simulink model "rudder_calibration"  (Simulink 7.5)
settings: Solver=FixedStepDiscrete  SolverMode=SingleTasking  StartTime=0.0  StopTime=10.0  FixedStep=0.01  RelTol=1e-3
InitFcn:
  | boat_constants
undefined symbols (not defined in the file): DiscIntNeverNeededParam, enableHil, getSensorData, Init_onlyOnce, Init_Reset, initUart2, OC2max, processNewCommData, T_step, u1, uart2EnqueueActuatorData, y1
libraries: dsPICdrivers x14, simulink x8
settings Model: Creator=Bryant  LastModifiedBy=Bryant
settings OptimizationCC: LifeSpan=1
settings HardwareCC: ProdBitPerInt=16  ProdEndianess=LittleEndian  ProdWordSize=16  ProdHWDeviceType=16-bit Generic
settings RTWCC: SystemTargetFile=dspic.tlc  MakeCommand=make_CreateMPLAB  TemplateMakefile=dspic_pic30_gcc.tmf  PostCodeGenCommand=dsPIC_Compile()  Description=Embedded Target for Microchip dsPIC (real-time)  ProcessScript=dspic_make_rtw_hook
settings RTWCC: CustomSource=|
  | ../../../../../ECAN_dspic/circBuffer.c
  | ../../clib/commProtocol.c
  | ../../clib/uart2.c
settings STFCustomTargetCC: IncludeMdlTerminateFcn=off  GeneratePreprocessorConditionals=Disable all  SupportNonInlinedSFcns=off  SystemTargetFile=dspic.tlc
settings ERTTargetCC: MultiwordLength=2048  ParMdlRefBuildCompliant=off  CompOptLevelCompliant=off  IncludeMdlTerminateFcn=off  GeneratePreprocessorConditionals=Disable all  CombineOutputUpdateFcns=off  ERTFirstTimeCompliant=off  ERTCustomFileBanners=off  SupportContinuousTime=on  ModelStepFunctionPrototypeControlCompliant=off  CPPClassGenCompliant=off  InlinedParameterPlacement=NonHierarchical  ERTSrcFileBannerTemplate=dsPIC_code_template.cgt  ERTHdrFileBannerTemplate=dsPIC_code_template.cgt  ERTDataSrcFileTemplate=dsPIC_code_template.cgt  ERTDataHdrFileTemplate=dsPIC_code_template.cgt  ERTCustomFileTemplate=dsPIC_main.tlc  ConvertIfToSwitch=off
settings CustomProperty: DataType=string  Value=C:\PROGRA~1\MATLAB\R2010a\bin\win64\gmake

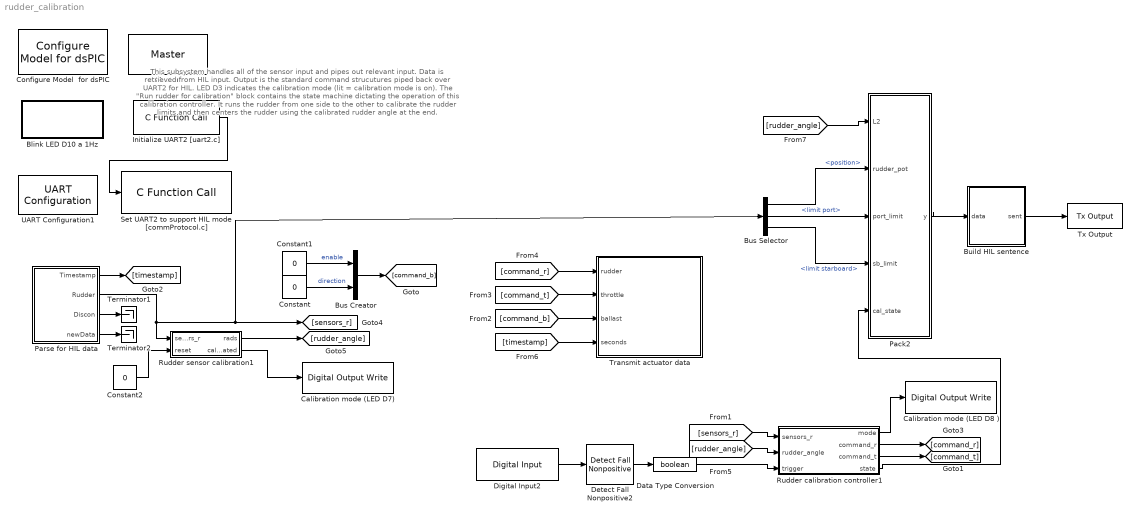
== system rudder_calibration ==
  note: This subsystem handles all of the sensor input and pipes out relevant input. Data is retrieved
      | from HIL input. Output is the standard command strucutures piped back over UART2 for HIL.
      | LED D3 indicates the calibration mode (lit = calibration mode is on).
      |
      | The "Run rudder for calibration" block contains the state machine dictating the operation of this
      | calibration controller. It runs the rudder from one side to the other to calibrate the rudder limits
      | and then centers the rudder using the calibrated rudder angle at the end.
  Blink LED D10 a 1Hz : Subsystem
      mask Display: disp('blink');
  Build HIL sentence : Subsystem
  Bus Creator : BusCreator  Inputs=2
  Bus Selector : BusSelector  OutputSignals=position,limit port,limit starboard
  Calibration mode (LED D7) : dsPICdrivers/Digital I//O/Digital Output Write  Tag=dsPIC_Digital_Output  Priority=5  PORT=A  Pin=[4]  Simultaneous=off  OrderingInOutPopup=None
  Calibration mode (LED D8 ) : dsPICdrivers/Digital I//O/Digital Output Write  Tag=dsPIC_Digital_Output  Priority=5  PORT=A  Pin=[5]  Simultaneous=off  OrderingInOutPopup=None
  Configure Model  for dsPIC : dsPICdrivers/Simulink Configuration/Configure Model  for dsPIC
  Constant : Constant  Value=0  OutDataTypeMode=boolean  OutDataType=fixdt(1, 16)  OutScaling=2^0  OutDataTypeStr=boolean
  Constant1 : Constant  Value=0  OutDataTypeMode=boolean  OutDataType=fixdt(1, 16)  OutScaling=2^0  OutDataTypeStr=boolean
  Constant2 : Constant  Value=0  OutDataTypeMode=boolean  OutDataType=fixdt(1, 16)  OutScaling=2^0  OutDataTypeStr=boolean
  Data Type Conversion : DataTypeConversion  OutDataTypeMode=boolean  OutDataType=fixdt(1, 16)  OutScaling=2^0  OutDataTypeStr=boolean
  Detect Fall Nonpositive2 : simulink/Logic and Bit Operations/Detect Fall Nonpositive  SystemSampleTime=-1  vinit=1
  Digital Input2 : dsPICdrivers/Digital I//O/Digital Input  Tag=dsPIC_Digital_Input  PORT=D  Pin=[7]  SampleTime=T_step  OrderingInOutPopup=None
  Initialize UART2 [uart2.c] : dsPICdrivers/OTHERS/C Function Call  Tag=dsPIC_dsPIC_CFunctionCall  FctUpdate=None  fctName='initUart2'  INPUT_SIZE=1  INPUT1=--  INPUT2=--  INPUT3=--  OUTPUT_SIZE=1  OUTPUT1=--  SampleTime=Inf  InputType=[]  OutputType=[]  FctDeclaration=extern void initUart2();  FctCall=initUart2();  OrderingInOutPopup=Output  FctStart=Start Function (Call once and only once)  FctStart_Name=initUart2  FctStart_Declaration=inline extern void initUart2();  FctStart_Call=initUart2();  FctInit=None  FctInit_Name=Init_Reset  FctInit_Declaration=inline extern void Init_Reset();  FctInit_Call=Init_Reset();
  Master : dsPICdrivers/Master  Tag=dsPIC_MASTER  Priority=1  TimeStepType=Timer1  picType=33fJ256GP710  fcy=40000000  Quartz_33f=8e6  PLLActive_33f=on  fcyDesired_33f=40000000  tmr1="[8  49999  0]"  tmr1Info="Time Step : 0.01  ;   Error : 0%  PR1=49999"  tmr2345="[0  0  0  0  0  0  0  0]"  tmr2345cfg=[-1 -1 -1 -1 -1 -1 -1 -1]  IOautoConf=on  typePort="[ 0   0   0   0  10  10   0  10   0   0   0   0   0   0   0   0   0   0   0   0   0   0   0   0   0   0   0   0   0   0   0   0   0   0   0   0   0   0   0   0   0   0   0   0   0   0   0   0   0   0   0   0   0   0   0   9   0   0   0   0   0   0   0   0   0   0   0   0   0   0   0   0   0   0   0   0   0   0   0   0   0   0   4   5   0   0   0   0   0   0   0   0   0   0   0   0   0   0   0   0   0   0   0   0   0   0   0   0   0   0   0   0 ]"  TRIS="[ 65359  65535  65535  65535  65535  65535  65535 ]"  ADPCFG=8388608  MasterBusyPort=None  MasterOverloadPort=None  FOSC=Quartz (XT - HS)  ClockSwitchMonitor=Both disabled  TempProtection_33f=TEMP_ON  FPBOR=<empty>  PWRT=disable  MCLR=<empty>  ICD=ICS_PGD1  JTAGEN=JTAGEN_OFF  PowerSave=off  OverrideFcy=off  NewFcy=1e6  PR2345="[65535  65535  65535  65535  65535  65535  65535  65535]"
  Pack2 : Stateflow chart  TreatAsAtomicUnit=on
  Parse for HIL data : Subsystem
  Rudder calibration controller1 : Subsystem
  Rudder sensor calibration1 : Subsystem
  Set UART2 to support HIL mode [commProtocol.c] : dsPICdrivers/OTHERS/C Function Call  Tag=dsPIC_dsPIC_CFunctionCall  FctUpdate=None  fctName='enableHil'  INPUT_SIZE=1  INPUT1=--  INPUT2=--  INPUT3=--  OUTPUT_SIZE=1  OUTPUT1=--  SampleTime=.01  InputType=[]  OutputType=[]  FctDeclaration=extern void enableHil();  FctCall=enableHil();  OrderingInOutPopup=Input  FctStart=Start Function (Call once and only once)  FctStart_Name=enableHil  FctStart_Declaration=inline extern void enableHil();  FctStart_Call=enableHil();  FctInit=None  FctInit_Name=Init_Reset  FctInit_Declaration=inline extern void Init_Reset();  FctInit_Call=Init_Reset();
  Terminator1 : Terminator
  Terminator2 : Terminator
  Transmit actuator data : Subsystem  TreatAsAtomicUnit=on
  Tx Output : dsPICdrivers/Serial PORT/Tx Output  Tag=dsPIC_TX  Priority=5  UART=1  OrderingInOutPopup=None
  UART Configuration1 : dsPICdrivers/Serial PORT/UART Configuration  Tag=dsPIC_config_UART  Priority=2  UART=1  proposed_BAUD=115200  BAUD=115200  ALT_TX_RX=on  InterruptTxWhen=When Transmit Buffer is empty  TXInterruptPri=1  TxBufferSize=32  TXEN=on  InterruptRxWhen=When Receive Buffer is full (contain 4 characters)  RXInterruptPri=2  RxBufferSize=32  DoNotImplementRxInterrupt=off  DoNotImplementTxInterrupt=off  UxBRG=21  Info="UxBRG = 21   ||  Real Baud : 113636   ||  % error : -1.3573  ||  max 113.6364 Bytes / Step"  RealBaud=0  ERROR=-1.3573  BYTES_STEP=113.6364
  wires:
  Parse for HIL data/2(Rudder) -> Rudder sensor calibration1/1(sensors_r), [sensors_r], Bus Selector/1
  [command_r] -> Transmit actuator data/1(rudder)
  [command_t] -> Transmit actuator data/2(throttle)
  [command_b] -> Transmit actuator data/3(ballast)
  Constant/1 -> Bus Creator/2  "direction"
  Bus Creator/1 -> [command_b]
  Constant1/1 -> Bus Creator/1  "enable"
  Parse for HIL data/1(Timestamp) -> [timestamp]
  Parse for HIL data/3(Discon) -> Terminator1/1
  Parse for HIL data/4(newData) -> Terminator2/1
  Rudder sensor calibration1/1(rads) -> [rudder_angle]
  Initialize UART2 [uart2.c]/1 -> Set UART2 to support HIL mode [commProtocol.c]/1
  [rudder_angle] -> Rudder calibration controller1/2(rudder_angle)
  Digital Input2/1 -> Detect Fall Nonpositive2/1
  [sensors_r] -> Rudder calibration controller1/1(sensors_r)
  Rudder calibration controller1/2(command_r) -> [command_r]
  Rudder calibration controller1/3(command_t) -> [command_t]
  Detect Fall Nonpositive2/1 -> Data Type Conversion/1
  Rudder calibration controller1/1(mode) -> Calibration mode (LED D8 )/1
  Data Type Conversion/1 -> Rudder calibration controller1/3(trigger)
  Rudder sensor calibration1/2(calibrated) -> Calibration mode (LED D7)/1
  Constant2/1 -> Rudder sensor calibration1/2(reset)
  [timestamp] -> Transmit actuator data/4(seconds)
  Pack2/1(y) -> Build HIL sentence/1(data)
  Build HIL sentence/1(sent) -> Tx Output/1
  [rudder_angle] -> Pack2/1(L2)
  Bus Selector/1 -> Pack2/2(rudder_pot)  "<position>"
  Bus Selector/2 -> Pack2/3(port_limit)  "<limit port>"
  Bus Selector/3 -> Pack2/4(sb_limit)  "<limit starboard>"
  Rudder calibration controller1/4(state) -> Pack2/5(cal_state)

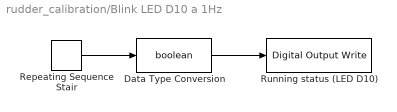
== system rudder_calibration/Blink LED D10 a 1Hz ==
  Data Type Conversion : DataTypeConversion  OutDataTypeMode=boolean  OutDataType=sfix(16)  OutScaling=2^0  OutDataTypeStr=boolean  RndMeth=Simplest
  Repeating Sequence Stair : simulink/Sources/Repeating Sequence Stair  SystemSampleTime=-1  OutValues=[1 0]  tsamp=1  OutMin=[]  OutMax=[]  OutDataTypeStr=double  OutputDataTypeScalingMode=double  OutDataType=fixdt(0,8)  ConRadixGroup=Best Precision: Vector-wise  OutScaling=2^-12
  Running status (LED D10) : dsPICdrivers/Digital I//O/Digital Output Write  Tag=dsPIC_Digital_Output  Priority=5  PORT=A  Pin=[7]  Simultaneous=off  OrderingInOutPopup=None
  wires:
  Repeating Sequence Stair/1 -> Data Type Conversion/1
  Data Type Conversion/1 -> Running status (LED D10)/1

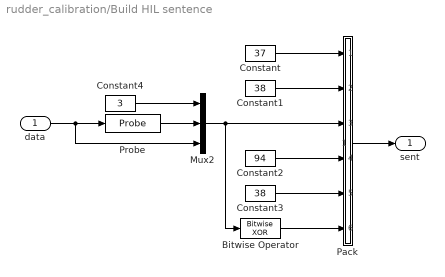
== system rudder_calibration/Build HIL sentence ==
  data : Inport
  Bitwise Operator : simulink/Logic and Bit Operations/Bitwise Operator  logicop=XOR  UseBitMask=off  BitMask=bin2dec('11011001')  BitMaskRealWorld=Stored Integer
  Constant : Constant  Value=37  OutDataTypeMode=uint8  OutDataType=fixdt(1, 16)  OutScaling=2^0  OutDataTypeStr=uint8
  Constant1 : Constant  Value=38  OutDataTypeMode=uint8  OutDataType=fixdt(1, 16)  OutScaling=2^0  OutDataTypeStr=uint8
  Constant2 : Constant  Value=94  OutDataTypeMode=uint8  OutDataType=fixdt(1, 16)  OutScaling=2^0  OutDataTypeStr=uint8
  Constant3 : Constant  Value=38  OutDataTypeMode=uint8  OutDataType=fixdt(1, 16)  OutScaling=2^0  OutDataTypeStr=uint8
  Constant4 : Constant  Value=3  OutDataTypeMode=uint8  OutDataType=fixdt(1, 16)  OutScaling=2^0  OutDataTypeStr=uint8
  Mux2 : Mux  Inputs=3
  Pack : Stateflow chart  TreatAsAtomicUnit=on
  Probe : Probe  ProbeSampleTime=off  ProbeComplexSignal=off  ProbeWidthDataType=uint8
  sent : Outport
  wires:
  data/1 -> Probe/1, Mux2/3
  Constant/1 -> Pack/1(a)
  Constant1/1 -> Pack/2(b)
  Pack/1(y) -> sent/1
  Mux2/1 -> Bitwise Operator/1, Pack/3(c)
  Probe/1 -> Mux2/2
  Constant2/1 -> Pack/4(d)
  Constant3/1 -> Pack/5(e)
  Bitwise Operator/1 -> Pack/6(f)
  Constant4/1 -> Mux2/1

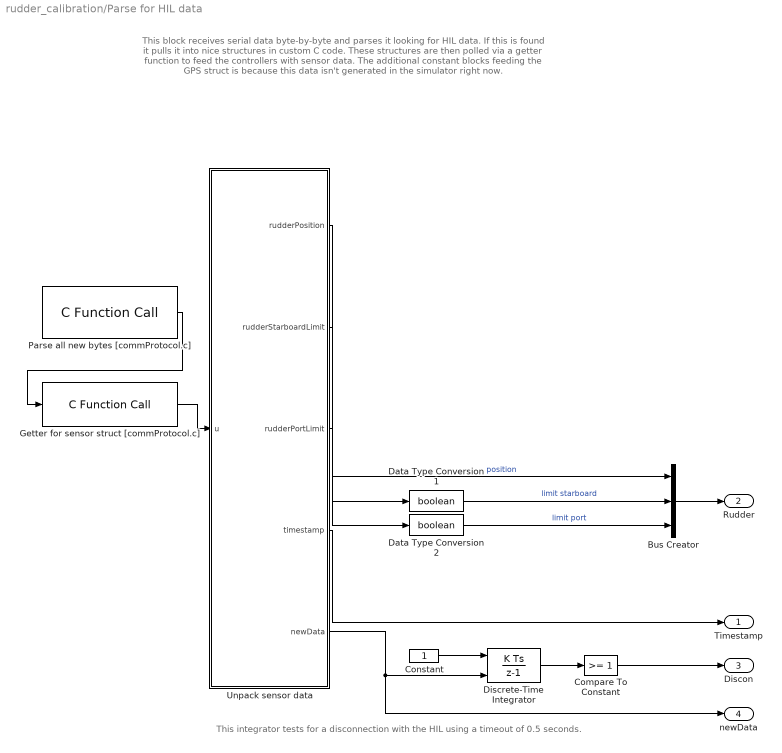
== system rudder_calibration/Parse for HIL data ==
  note: This block receives serial data byte-by-byte and parses it looking for HIL data.
      | If this is found it pulls it into nice structures in custom C code. These structures
      | are then polled via a getter function to feed the controllers with sensor data.
      |
      | The additional constant blocks feeding the GPS struct is because this data isn't
      | generated in the simulator right now.
  note: This integrator tests for a disconnection with the HIL
      | using a timeout of 0.5 seconds.
  Bus Creator : BusCreator  Inputs=3
  Compare To Constant : simulink/Logic and Bit Operations/Compare To Constant  SystemSampleTime=-1  relop=>=  const=1  LogicOutDataTypeMode=boolean
  Constant : Constant  OutDataTypeMode=uint8  OutDataType=fixdt(1, 16)  OutScaling=2^0  OutDataTypeStr=uint8
  Data Type Conversion1 : DataTypeConversion  OutDataTypeMode=boolean  OutDataType=fixdt(1, 16)  OutScaling=2^0  OutDataTypeStr=boolean
  Data Type Conversion2 : DataTypeConversion  OutDataTypeMode=boolean  OutDataType=fixdt(1, 16)  OutScaling=2^0  OutDataTypeStr=boolean
  Discrete-Time Integrator : DiscreteIntegrator  gainval=2  ExternalReset=level  SampleTime=T_step  OutDataType=fixdt(1, 16)  OutScaling=2^0  LimitOutput=on  UpperSaturationLimit=1  LowerSaturationLimit=0  ICPrevOutput=DiscIntNeverNeededParam  ICPrevScaledInput=DiscIntNeverNeededParam
  Getter for sensor struct [commProtocol.c] : dsPICdrivers/OTHERS/C Function Call  Tag=dsPIC_dsPIC_CFunctionCall  FctUpdate=Output Function  fctName='getSensorData'  INPUT_SIZE=1  INPUT1=--  INPUT2=--  INPUT3=--  OUTPUT_SIZE=40  OUTPUT1=uint8  SampleTime=.01  InputType=[ ]  OutputType=[ 2 ]  FctDeclaration=extern void getSensorData(uint8_T* y1);  FctCall=getSensorData(*%y1);  OrderingInOutPopup=Input  FctStart=None  FctStart_Name=Init_onlyOnce  FctStart_Declaration=inline extern void Init_onlyOnce();  FctStart_Call=Init_onlyOnce();  FctInit=None  FctInit_Name=Init_Reset  FctInit_Declaration=inline extern void Init_Reset();  FctInit_Call=Init_Reset();
  Parse all new bytes [commProtocol.c] : dsPICdrivers/OTHERS/C Function Call  Tag=dsPIC_dsPIC_CFunctionCall  FctUpdate=Output Function  fctName='processNewCommData'  INPUT_SIZE=1  INPUT1=--  INPUT2=--  INPUT3=--  OUTPUT_SIZE=1  OUTPUT1=--  SampleTime=.01  InputType=[ ]  OutputType=[ ]  FctDeclaration=extern void processNewCommData();  FctCall=processNewCommData();  OrderingInOutPopup=Output  FctStart=None  FctStart_Name=Init_onlyOnce  FctStart_Declaration=inline extern void Init_onlyOnce();  FctStart_Call=Init_onlyOnce();  FctInit=None  FctInit_Name=Init_Reset  FctInit_Declaration=inline extern void Init_Reset();  FctInit_Call=Init_Reset();
  Unpack sensor data : Stateflow chart  TreatAsAtomicUnit=on
  Timestamp : Outport
  Rudder : Outport  Port=2
  Discon : Outport  Port=3
  newData : Outport  Port=4
  wires:
  Bus Creator/1 -> Rudder/1
  Getter for sensor struct [commProtocol.c]/1 -> Unpack sensor data/1(u)
  Parse all new bytes [commProtocol.c]/1 -> Getter for sensor struct [commProtocol.c]/1
  Unpack sensor data/1(rudderPosition) -> Bus Creator/1  "position"
  Unpack sensor data/2(rudderStarboardLimit) -> Data Type Conversion1/1
  Unpack sensor data/3(rudderPortLimit) -> Data Type Conversion2/1
  Unpack sensor data/4(timestamp) -> Timestamp/1
  Constant/1 -> Discrete-Time Integrator/1
  Discrete-Time Integrator/1 -> Compare To Constant/1
  Unpack sensor data/5(newData) -> Discrete-Time Integrator/2, newData/1
  Compare To Constant/1 -> Discon/1
  Data Type Conversion1/1 -> Bus Creator/2  "limit starboard"
  Data Type Conversion2/1 -> Bus Creator/3  "limit port"

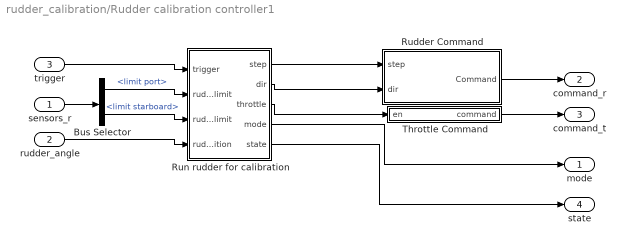
== system rudder_calibration/Rudder calibration controller1 ==
  sensors_r : Inport
  rudder_angle : Inport  Port=2
  trigger : Inport  Port=3
  Bus Selector : BusSelector  OutputSignals=limit port,limit starboard
  Rudder Command : Subsystem
  Run rudder for calibration : Stateflow chart  TreatAsAtomicUnit=on
  Throttle Command : Subsystem
  mode : Outport
  command_r : Outport  Port=2
  command_t : Outport  Port=3
  state : Outport  Port=4
  wires:
  trigger/1 -> Run rudder for calibration/1(trigger)
  Bus Selector/1 -> Run rudder for calibration/2(rudder_port_limit)  "<limit port>"
  Bus Selector/2 -> Run rudder for calibration/3(rudder_sb_limit)  "<limit starboard>"
  Run rudder for calibration/1(step) -> Rudder Command/1(step)
  Run rudder for calibration/2(dir) -> Rudder Command/2(dir)
  Run rudder for calibration/3(throttle) -> Throttle Command/1(en)
  sensors_r/1 -> Bus Selector/1
  rudder_angle/1 -> Run rudder for calibration/4(rudder_position)
  Throttle Command/1(command) -> command_t/1
  Rudder Command/1(Command) -> command_r/1
  Run rudder for calibration/4(mode) -> mode/1
  Run rudder for calibration/5(state) -> state/1

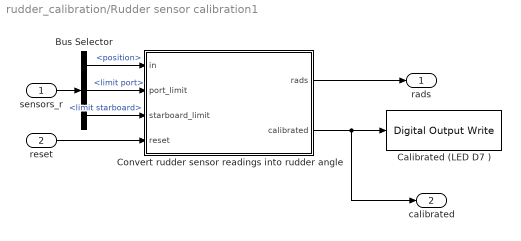
== system rudder_calibration/Rudder sensor calibration1 ==
  sensors_r : Inport
  reset : Inport  Port=2
  Bus Selector : BusSelector  OutputSignals=position,limit port,limit starboard
  Calibrated (LED D7 ) : dsPICdrivers/Digital I//O/Digital Output Write  Tag=dsPIC_Digital_Output  Priority=5  PORT=A  Pin=[4]  Simultaneous=off  OrderingInOutPopup=None
  Convert rudder sensor readings into rudder angle : Stateflow chart  TreatAsAtomicUnit=on
  rads : Outport
  calibrated : Outport  Port=2
  wires:
  Convert rudder sensor readings into rudder angle/1(rads) -> rads/1
  sensors_r/1 -> Bus Selector/1
  Bus Selector/1 -> Convert rudder sensor readings into rudder angle/1(in)  "<position>"
  Bus Selector/2 -> Convert rudder sensor readings into rudder angle/2(port_limit)  "<limit port>"
  Bus Selector/3 -> Convert rudder sensor readings into rudder angle/3(starboard_limit)  "<limit starboard>"
  Convert rudder sensor readings into rudder angle/2(calibrated) -> Calibrated (LED D7 )/1, calibrated/1
  reset/1 -> Convert rudder sensor readings into rudder angle/4(reset)

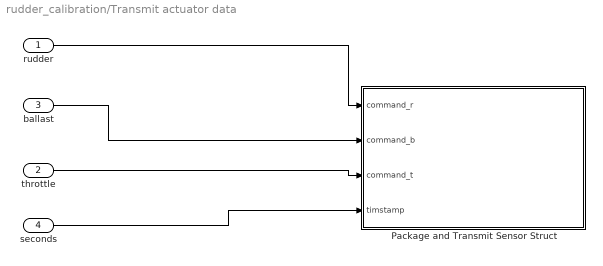
== system rudder_calibration/Transmit actuator data ==
  rudder : Inport  OutDataType=fixdt(1, 16)  OutScaling=2^0
  throttle : Inport  Port=2  OutDataType=fixdt(1, 16)  OutScaling=2^0
  ballast : Inport  Port=3  OutDataType=fixdt(1, 16)  OutScaling=2^0
  seconds : Inport  Port=4  OutDataType=fixdt(1, 16)  OutScaling=2^0
  Package and Transmit Sensor Struct : Subsystem
  wires:
  rudder/1 -> Package and Transmit Sensor Struct/1(command_r)
  throttle/1 -> Package and Transmit Sensor Struct/3(command_t)
  ballast/1 -> Package and Transmit Sensor Struct/2(command_b)
  seconds/1 -> Package and Transmit Sensor Struct/4(timstamp)

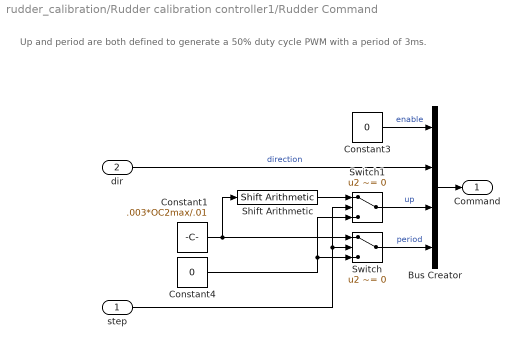
== system rudder_calibration/Rudder calibration controller1/Rudder Command ==
  note: Up and period are both defined to generate a 50% duty cycle PWM with
      | a period of 3ms.
  step : Inport
  dir : Inport  Port=2
  Bus Creator : BusCreator
  Constant1 : Constant  Value=.003*OC2max/.01  OutDataTypeMode=uint16  OutDataType=sfix(16)  OutScaling=2^0  OutDataTypeStr=uint16
  Constant3 : Constant  Value=0  OutDataTypeMode=boolean  OutDataType=sfix(16)  OutScaling=2^0  OutDataTypeStr=boolean
  Constant4 : Constant  Value=0  OutDataTypeMode=uint16  OutDataType=sfix(16)  OutScaling=2^0  OutDataTypeStr=uint16
  Shift Arithmetic : simulink/Logic and Bit Operations/Shift Arithmetic  SystemSampleTime=-1  nBitShiftRight=1  nBinPtShiftRight=0
  Switch : Switch  Criteria=u2 ~= 0  OutDataType=fixdt(1, 16)  OutScaling=2^0
  Switch1 : Switch  Criteria=u2 ~= 0  OutDataType=fixdt(1, 16)  OutScaling=2^0
  Command : Outport
  wires:
  step/1 -> Switch1/2, Switch/2
  Constant4/1 -> Switch1/3, Switch/3
  Switch1/1 -> Bus Creator/3  "up"
  Switch/1 -> Bus Creator/4  "period"
  Shift Arithmetic/1 -> Switch1/1
  Constant1/1 -> Switch/1, Shift Arithmetic/1
  Constant3/1 -> Bus Creator/1  "enable"
  Bus Creator/1 -> Command/1
  dir/1 -> Bus Creator/2  "direction"

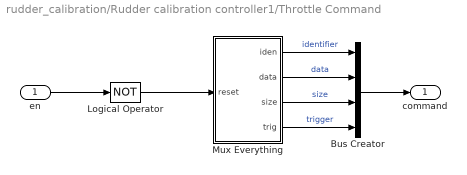
== system rudder_calibration/Rudder calibration controller1/Throttle Command ==
  en : Inport
  Bus Creator : BusCreator
  Logical Operator : Logic  Operator=NOT  AllPortsSameDT=off  OutDataTypeMode=boolean  LogicDataType=fixdt(0, 8)  OutDataTypeStr=boolean
  Mux Everything : Subsystem
  command : Outport  OutDataType=sfix(16)  OutScaling=2^0
  wires:
  Mux Everything/3(size) -> Bus Creator/3  "size"
  Mux Everything/2(data) -> Bus Creator/2  "data"
  Mux Everything/1(iden) -> Bus Creator/1  "identifier"
  en/1 -> Logical Operator/1
  Bus Creator/1 -> command/1
  Logical Operator/1 -> Mux Everything/1(reset)
  Mux Everything/4(trig) -> Bus Creator/4  "trigger"

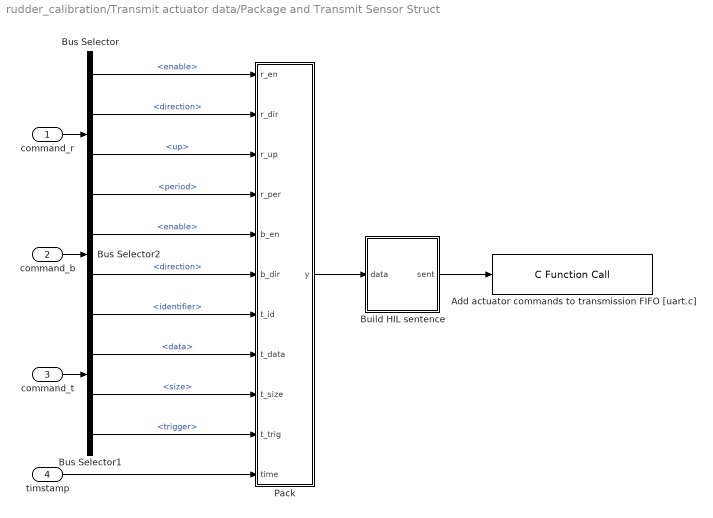
== system rudder_calibration/Transmit actuator data/Package and Transmit Sensor Struct ==
  command_r : Inport
  command_b : Inport  Port=2
  command_t : Inport  Port=3
  timstamp : Inport  Port=4
  Add actuator commands to transmission FIFO [uart.c] : dsPICdrivers/OTHERS/C Function Call  Tag=dsPIC_dsPIC_CFunctionCall  FctUpdate=Output Function  fctName='uart2EnqueueActuatorData'  INPUT_SIZE=29  INPUT1=uint8  INPUT2=--  INPUT3=--  OUTPUT_SIZE=1  OUTPUT1=--  SampleTime=-1  InputType=[ 2 ]  OutputType=[ ]  FctDeclaration=extern void uart2EnqueueActuatorData(uint8_T* u1);  FctCall=uart2EnqueueActuatorData(*%u1);  OrderingInOutPopup=None  FctStart=None  FctStart_Name=Init_onlyOnce  FctStart_Declaration=inline extern void Init_onlyOnce();  FctStart_Call=Init_onlyOnce();  FctInit=None  FctInit_Name=Init_Reset  FctInit_Declaration=inline extern void Init_Reset();  FctInit_Call=Init_Reset();
  Build HIL sentence : Subsystem
  Bus Selector : BusSelector  OutputSignals=enable,direction,up,period
  Bus Selector1 : BusSelector  OutputSignals=identifier,data,size,trigger
  Bus Selector2 : BusSelector  OutputSignals=enable,direction
  Pack : Stateflow chart  TreatAsAtomicUnit=on
  wires:
  Bus Selector/2 -> Pack/2(r_dir)  "<direction>"
  Bus Selector/1 -> Pack/1(r_en)  "<enable>"
  Bus Selector1/4 -> Pack/10(t_trig)  "<trigger>"
  Bus Selector/3 -> Pack/3(r_up)  "<up>"
  Bus Selector2/1 -> Pack/5(b_en)  "<enable>"
  Bus Selector/4 -> Pack/4(r_per)  "<period>"
  Bus Selector1/2 -> Pack/8(t_data)  "<data>"
  Bus Selector1/3 -> Pack/9(t_size)  "<size>"
  command_r/1 -> Bus Selector/1
  command_b/1 -> Bus Selector2/1
  command_t/1 -> Bus Selector1/1
  timstamp/1 -> Pack/11(time)
  Build HIL sentence/1(sent) -> Add actuator commands to transmission FIFO [uart.c]/1
  Pack/1(y) -> Build HIL sentence/1(data)
  Bus Selector2/2 -> Pack/6(b_dir)  "<direction>"
  Bus Selector1/1 -> Pack/7(t_id)  "<identifier>"

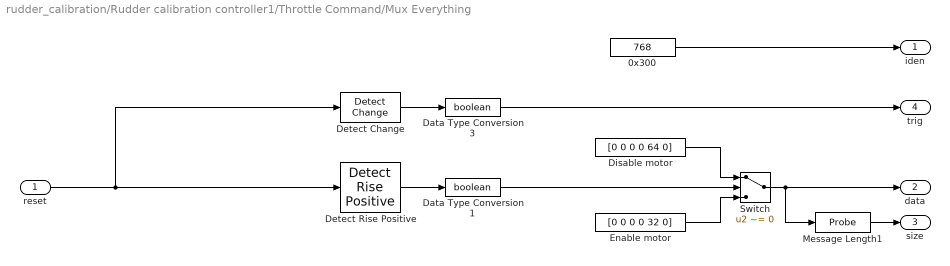
== system rudder_calibration/Rudder calibration controller1/Throttle Command/Mux Everything ==
  reset : Inport  OutDataType=sfix(16)  OutScaling=2^0
  0x300 : Constant  Value=768  OutDataTypeMode=uint32  OutDataType=sfix(16)  OutScaling=2^0  OutDataTypeStr=uint32
  Data Type Conversion1 : DataTypeConversion  OutDataTypeMode=boolean  OutDataType=sfix(16)  OutScaling=2^0  OutDataTypeStr=boolean
  Data Type Conversion3 : DataTypeConversion  OutDataTypeMode=boolean  OutDataType=sfix(16)  OutScaling=2^0  OutDataTypeStr=boolean
  Detect Change : simulink/Logic and Bit Operations/Detect Change  SystemSampleTime=-1  vinit=0
  Detect Rise Positive : simulink/Logic and Bit Operations/Detect Rise Positive  SystemSampleTime=-1  vinit=0
  Disable motor : Constant  Value=[0 0 0 0 64 0]  OutDataTypeMode=uint8  OutDataType=sfix(16)  OutScaling=2^0  OutDataTypeStr=uint8
  Enable motor : Constant  Value=[0 0 0 0 32 0]  OutDataTypeMode=uint8  OutDataType=sfix(16)  OutScaling=2^0  OutDataTypeStr=uint8
  Message Length1 : Probe  ProbeSampleTime=off  ProbeComplexSignal=off  ProbeWidthDataType=uint8
  Switch : Switch  Criteria=u2 ~= 0  OutDataType=fixdt(1, 16)  OutScaling=2^0
  iden : Outport  OutDataType=sfix(16)  OutScaling=2^0
  data : Outport  Port=2  OutDataType=sfix(16)  OutScaling=2^0
  size : Outport  Port=3  OutDataType=sfix(16)  OutScaling=2^0
  trig : Outport  Port=4  OutDataType=sfix(16)  OutScaling=2^0
  wires:
  0x300/1 -> iden/1
  Message Length1/1 -> size/1
  Switch/1 -> data/1, Message Length1/1
  Disable motor/1 -> Switch/1
  Enable motor/1 -> Switch/3
  Data Type Conversion1/1 -> Switch/2
  Detect Rise Positive/1 -> Data Type Conversion1/1
  reset/1 -> Detect Rise Positive/1, Detect Change/1
  Detect Change/1 -> Data Type Conversion3/1
  Data Type Conversion3/1 -> trig/1

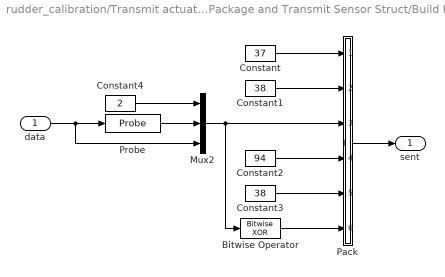
== system rudder_calibration/Transmit actuator data/Package and Transmit Sensor Struct/Build HIL sentence ==
  data : Inport
  Bitwise Operator : simulink/Logic and Bit Operations/Bitwise Operator  logicop=XOR  UseBitMask=off  BitMask=bin2dec('11011001')  BitMaskRealWorld=Stored Integer
  Constant : Constant  Value=37  OutDataTypeMode=uint8  OutDataType=fixdt(1, 16)  OutScaling=2^0  OutDataTypeStr=uint8
  Constant1 : Constant  Value=38  OutDataTypeMode=uint8  OutDataType=fixdt(1, 16)  OutScaling=2^0  OutDataTypeStr=uint8
  Constant2 : Constant  Value=94  OutDataTypeMode=uint8  OutDataType=fixdt(1, 16)  OutScaling=2^0  OutDataTypeStr=uint8
  Constant3 : Constant  Value=38  OutDataTypeMode=uint8  OutDataType=fixdt(1, 16)  OutScaling=2^0  OutDataTypeStr=uint8
  Constant4 : Constant  Value=2  OutDataTypeMode=uint8  OutDataType=fixdt(1, 16)  OutScaling=2^0  OutDataTypeStr=uint8
  Mux2 : Mux  Inputs=3
  Pack : Stateflow chart  TreatAsAtomicUnit=on
  Probe : Probe  ProbeSampleTime=off  ProbeComplexSignal=off  ProbeWidthDataType=uint8
  sent : Outport
  wires:
  data/1 -> Probe/1, Mux2/3
  Constant/1 -> Pack/1(a)
  Constant1/1 -> Pack/2(b)
  Pack/1(y) -> sent/1
  Mux2/1 -> Bitwise Operator/1, Pack/3(c)
  Probe/1 -> Mux2/2
  Constant2/1 -> Pack/4(d)
  Constant3/1 -> Pack/5(e)
  Bitwise Operator/1 -> Pack/6(f)
  Constant4/1 -> Mux2/1

== matlab function Rudder sensor calibration1/Convert rudder sensor readings into rudder angle ==
  data: in input uint16; rads output single; port_limit input boolean; starboard_limit input boolean; calibrated output double; reset input double
function [rads, calibrated] = pot_to_rads(in, port_limit, starboard_limit, reset)
%#eml

persistent low_side high_side lastInput offset cal
if isempty(low_side) || isempty(high_side) || reset
    low_side = int32(-1);
    high_side = int32(-1);
    lastInput = int32(-10000);
    offset = int32(0);
    cal = false;
end

% Here we track transitions. On a high->low transition start adding 1023
% and on a low->high transition don't add anything. It "centers" the input
% range around 1023.
input = int32(in);
if lastInput == uint32(-10000)
    lastInput = input;
end
jump = input - lastInput;
if jump > 1000
    offset = int32(0);
elseif jump < -1000
    offset = int32(1023);
end

% We record the last input BEFORE it's offset. This fixes situations where
% we're comparing data before and after the very first transition.
lastInput = input;

% Apply any offset that should be there.
input = input + offset;

% Update port range limit when the Hall limit switch. Only update to the
% maximum value obtained during the limit switch active period.
if port_limit && high_side == -1
    high_side = input;
    
    % If the high_side limit is less than the low_side one, we add 1023
    % assuming that it's a valid value (ie. ~= -1).
    if high_side < low_side && high_side ~= -1
        high_side = high_side + 1023;
    end
    
    if low_side ~= -1
        cal = true;
    end
end

% Update starboard ADC value when limit is reached. Only update to the
% maximum value obtained during the limit switch active period.
if starboard_limit && low_side == -1
    low_side = input;
    
    % If the high_side limit is less than the low_side one, we add 1023
    % assuming that it's a valid value (ie. ~= -1).
    if high_side < low_side && high_side ~= -1
        high_side = high_side + 1023;
    end
    
    if high_side ~= -1
        cal = true;
    end
end

calibrated = cal;

% Return 0 when we can't actually determine the rudder position
if ~cal
    rads = single(0);
    return;
end

% Prepare our input. Here we subtract the baseline 'low_side' value off of
% the input so we start with a range from [0..high_side-lowside] and map it
% into the output range of 45 degrees.
in_min = 0;
in_max = high_side - low_side;
out_min = int32(-45);
out_max = int32(45);
val = input - low_side;

% This is a basic integer implementation of a map() function. It was pulled
% from: http://www.arduino.cc/cgi-bin/yabb2/YaBB.pl?num=1289758376, first
% post.
% NOTE: There can be integer overflow in the first multiplication, but with
% the set of inputs we're seeing here the maximum value of the multiplication
% is 90*1023 = 92070, far below intmax32.
mappedValue = (val - in_min) * (out_max - out_min) / (in_max - in_min) + out_min;

% Finally convert to radians and a double before returning it.
rads = single(mappedValue) * pi / 180;

== matlab function Transmit actuator data/Package and Transmit Sensor Struct/Pack ==
  data: r_en input double; y output uint8 size=22; r_dir input double; r_up input double; r_per input double; b_en input double; b_dir input double; t_id input uint32; t_data input double; t_size input double; t_trig input double; time input double
function y = fcn(r_en, r_dir, r_up, r_per, b_en, b_dir, t_id, t_data, t_size, t_trig, time)
%#eml

y = zeros(22, 1, 'uint8');
y(1) = uint8(r_en);
y(2) = uint8(r_dir);
y(3) = uint8(bitand(r_up,hex2dec('FF')));
y(4) = uint8(bitand(bitshift(r_up,-8),hex2dec('FF')));
y(5) = uint8(bitand(r_per,hex2dec('FF')));
y(6) = uint8(bitand(bitshift(r_per,-8),hex2dec('FF')));
y(7) = uint8(b_en);
y(8) = uint8(b_dir);
tid_cast = typecast(t_id, 'uint32');
y(9) = uint8(bitand(tid_cast,hex2dec('FF')));
y(10) = uint8(bitand(bitshift(tid_cast,-8),hex2dec('FF')));
y(11) = uint8(bitand(bitshift(tid_cast,-16),hex2dec('FF')));
y(12) = uint8(bitand(bitshift(tid_cast,-24),hex2dec('FF')));
y(13:18) = t_data(1:6);
y(19) = t_size;
y(20) = uint8(t_trig);
y(21) = uint8(bitand(typecast(time,'uint16'),hex2dec('FF')));
y(22) = uint8(bitand(bitshift(typecast(time,'uint16'),-8),hex2dec('FF')));

== matlab function Transmit actuator data/Package and Transmit Sensor Struct/Build HIL sentence/Pack ==
  data: a input double; y output double; b input double; c input double; d input double; e input double; f input double
function y = fcn(a, b, c, d, e, f)
%#eml

y = zeros(29, 1, 'uint8');
y(1) = a;
y(2) = b;
y(3:26) = c;
y(27) = d;
y(28) = e;
y(29) = f;

== matlab function Rudder calibration controller1/Run rudder for calibration ==
  data: trigger input double; step output double; rudder_port_limit input double; rudder_sb_limit input double; dir output double; throttle output double; rudder_position input double; mode output double; state output double
function [step, dir, throttle, mode, state] = calibrate(trigger, rudder_port_limit, rudder_sb_limit, rudder_position)
%#eml

% cal_state stores which state we're in. 0 indicates no calibration, 2 means
% calibrating the port limit, 1 means calibration the starboard limit
persistent cal_state direction run drive cal_mode
if isempty(cal_state)
    cal_state = uint8(0);
    direction = false;
    run = false;
    cal_mode = false;
    drive = true; % Drive is initialized to true here such that it will trigger a transition at the start and end of the calibration control code.
end

if trigger
    cal_mode = ~cal_mode;
end

mode = cal_mode;

if cal_state == 0 % Waiting for calibration trigger
    if trigger
        cal_state = uint8(6);
        drive = false;
    end
elseif cal_state == 6 % Initial calibration mode
    if ~cal_mode % Reset if calibration is disabled
        cal_state = uint8(0);
        run = false;
        drive = true;
    elseif rudder_sb_limit % If the starboard limit is active, go to port first
        cal_state = uint8(5);
        run = true;
        direction = true;
    else % Default to running to starboard first
        cal_state = uint8(4);
        run = true;
        direction = false;
    end
elseif cal_state == 5 % Calibrating the first limit (port)
    if ~cal_mode % Reset if calibration is disabled
        cal_state = uint8(0);
        run = false;
        drive = true;
    elseif rudder_port_limit % If we've hit the limit, we're done here
        cal_state = uint8(2);
        direction = false;
    end
elseif cal_state == 4 % Calibrating the first limit (starboard)
    if ~cal_mode % Reset if calibration is disabled
        cal_state = uint8(0);
        run = false;
        drive = true;
    elseif rudder_sb_limit % If we've hit the limit, we're done here
        cal_state = uint8(3);
        direction = true;
    end
elseif cal_state == 3 % Last limit calibration (port)
    if ~cal_mode % Reset if calibration is disabled
        cal_state = uint8(0);
        run = false;
        drive = true;
    elseif rudder_port_limit % If we've hit the port limit then we're done calibrating, so we recenter the rudder.
        cal_state = uint8(1);
        direction = false;
    end
elseif cal_state == 2 % Last limit calibration (starboard)
    if ~cal_mode % Reset if calibration is disabled
        cal_state = uint8(0);
        run = false;
        drive = true;
    elseif rudder_sb_limit % If we've hit the starboard limit then we're done calibrating, so we recenter the rudder.
        cal_state = uint8(1);
        direction = true;
    end
elseif cal_state == 1 % Center the rudder
    if ~cal_mode % Reset if calibration is disabled
        cal_state = uint8(0);
        run = false;
        drive = true;
    elseif abs(rudder_position) < 0.03 % If we've reached the center, then we're all done!
        cal_state = uint8(0);
        run = false;
        drive = true;
        cal_mode = false;
    end
end

state = cal_state;
step = run;
dir = direction;
throttle = drive;

== matlab function Parse for HIL data/Unpack sensor data ==
  data: u input uint8; rudderPosition output double; rudderStarboardLimit output double; rudderPortLimit output double; timestamp output double; newData output double
function [rudderPosition, rudderStarboardLimit, rudderPortLimit, timestamp, newData] = unpack(u)
%#eml

rudderPosition = typecast(u(30:31), 'uint16');
rudderStarboardLimit = u(32);
rudderPortLimit = u(33);
timestamp = typecast(u(38:39), 'int16');
newData = u(40);

== matlab function Pack2 ==
  data: L2 input double; y output double; rudder_pot input double; port_limit input double; sb_limit input double; cal_state input double
function y = fcn(L2, rudder_pot, port_limit, sb_limit, cal_state)
%#eml

y = zeros(90, 1, 'uint8');
y(1:4) = packUint32BE(typecast(L2,'uint32'));
y(53:54) = packUint16BE(rudder_pot);
y(55) = port_limit;
y(56) = sb_limit;
y(88) = cal_state;

function out = packUint32BE(in)
out = zeros(4, 1, 'uint8');
out(1) = uint8(bitand(bitshift(in,-24),hex2dec('FF')));
out(2) = uint8(bitand(bitshift(in,-16),hex2dec('FF')));
out(3) = uint8(bitand(bitshift(in,-8),hex2dec('FF')));
out(4) = uint8(bitand(in,hex2dec('FF')));

function out = packUint16BE(in)
out = zeros(2, 1, 'uint8');
out(1) = uint8(bitand(bitshift(in,-8),hex2dec('FF')));
out(2) = uint8(bitand(in,hex2dec('FF')));

== matlab function Build HIL sentence/Pack ==
  data: a input double; y output double; b input double; c input double; d input double; e input double; f input double
function y = fcn(a, b, c, d, e, f)
%#eml

y = zeros(length(a)+length(b)+length(c)+length(d)+length(e)+length(f), 1, 'uint8');
y(1) = a;
y(2) = b;
y(3:94) = c;
y(95) = d;
y(96) = e;
y(97) = f;
